simulink model "ctrl_student"  (R2014a)
settings: Solver=ode4  StartTime=0.0  StopTime=inf  FixedStep=0.01  RelTol=1e-3
undefined symbols (not defined in the file): M
libraries: marine_gnc x2
(part 2 of 2)

== system ctrl_student/Observer/nu_hat ==
  nu_hat : Inport
  Demux : Demux  Outputs=3
  r_hat : S-Function  Priority=3  FunctionName=NIVeriStandIO  Parameters=width dtype portnum stime stype btype  EnableBusSupport=off  mask(NI VeriStand Outport){portnum=3, width=-1, stime=-1, dtype=auto, stype=auto, btype=0}
      mask prompts: portnum "Port number:"; width "Port dimensions (-1 for dynamically sized):"; stime "Sample time (-1 for inherited):"; dtype "Data type:"; stype "Signal type:"; btype "Block type:"
      mask help: Use this outport on any level of nested subsystems to allow NI VeriStand software to map signals to it.
      mask init:
      | NIVeriStandIO_init;
      settings: CopyFcn=NIVeriStand_MDL_functions('', 'IO_copy');  DeleteFcn=NIVeriStand_MDL_functions('', 'IO_delete');  MoveFcn=set_param(gcb, 'Mask', 'on');
      mask Callback portnum: NIVeriStand_MDL_functions('', 'IO_setportnum');
      mask TypeOptions dtype: auto | double | single | int8 | uint8 | int16 | uint16 | int32 | uint32 | boolean
      mask Callback dtype: NIVeriStand_MDL_functions('', 'IO_booleansignal');
      mask TypeOptions stype: auto | real | complex
      mask Display:
      | patch([-x x], [-y y], [.90980 .81960 .32156]);
      | plot([xrad -x x xrad], [yrad -y y yrad]);
      | fprintf('NI Out%d', portnum);
  u_hat : S-Function  Priority=1  FunctionName=NIVeriStandIO  Parameters=width dtype portnum stime stype btype  EnableBusSupport=off  mask(NI VeriStand Outport){portnum=1, width=-1, stime=-1, dtype=auto, stype=auto, btype=0}
      mask prompts: portnum "Port number:"; width "Port dimensions (-1 for dynamically sized):"; stime "Sample time (-1 for inherited):"; dtype "Data type:"; stype "Signal type:"; btype "Block type:"
      mask help: Use this outport on any level of nested subsystems to allow NI VeriStand software to map signals to it.
      mask init:
      | NIVeriStandIO_init;
      settings: CopyFcn=NIVeriStand_MDL_functions('', 'IO_copy');  DeleteFcn=NIVeriStand_MDL_functions('', 'IO_delete');  MoveFcn=set_param(gcb, 'Mask', 'on');
      mask Callback portnum: NIVeriStand_MDL_functions('', 'IO_setportnum');
      mask TypeOptions dtype: auto | double | single | int8 | uint8 | int16 | uint16 | int32 | uint32 | boolean
      mask Callback dtype: NIVeriStand_MDL_functions('', 'IO_booleansignal');
      mask TypeOptions stype: auto | real | complex
      mask Display:
      | patch([-x x], [-y y], [.90980 .81960 .32156]);
      | plot([xrad -x x xrad], [yrad -y y yrad]);
      | fprintf('NI Out%d', portnum);
  v_hat : S-Function  Priority=2  FunctionName=NIVeriStandIO  Parameters=width dtype portnum stime stype btype  EnableBusSupport=off  mask(NI VeriStand Outport){portnum=2, width=-1, stime=-1, dtype=auto, stype=auto, btype=0}
      mask prompts: portnum "Port number:"; width "Port dimensions (-1 for dynamically sized):"; stime "Sample time (-1 for inherited):"; dtype "Data type:"; stype "Signal type:"; btype "Block type:"
      mask help: Use this outport on any level of nested subsystems to allow NI VeriStand software to map signals to it.
      mask init:
      | NIVeriStandIO_init;
      settings: CopyFcn=NIVeriStand_MDL_functions('', 'IO_copy');  DeleteFcn=NIVeriStand_MDL_functions('', 'IO_delete');  MoveFcn=set_param(gcb, 'Mask', 'on');
      mask Callback portnum: NIVeriStand_MDL_functions('', 'IO_setportnum');
      mask TypeOptions dtype: auto | double | single | int8 | uint8 | int16 | uint16 | int32 | uint32 | boolean
      mask Callback dtype: NIVeriStand_MDL_functions('', 'IO_booleansignal');
      mask TypeOptions stype: auto | real | complex
      mask Display:
      | patch([-x x], [-y y], [.90980 .81960 .32156]);
      | plot([xrad -x x xrad], [yrad -y y yrad]);
      | fprintf('NI Out%d', portnum);
  wires:
  Demux/1 -> u_hat/1
  Demux/2 -> v_hat/1
  Demux/3 -> r_hat/1
  nu_hat/1 -> Demux/1

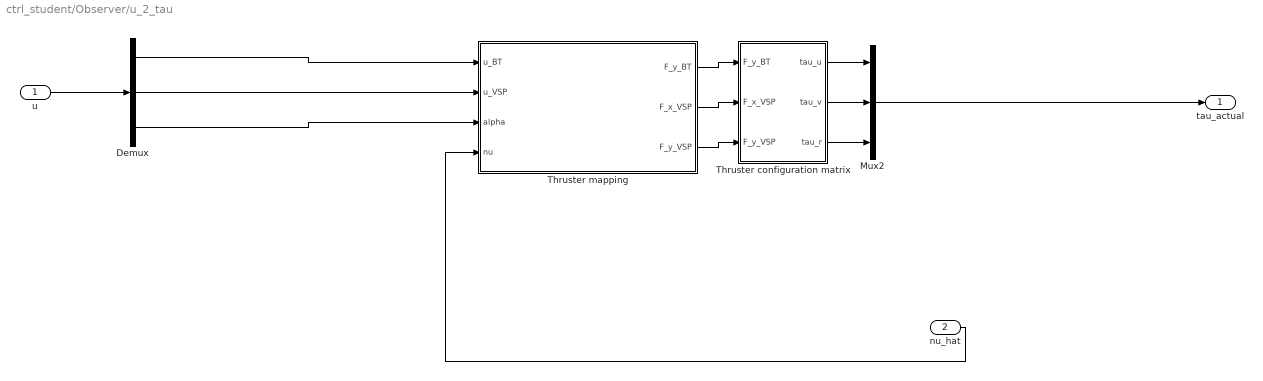
== system ctrl_student/Observer/u_2_tau ==
  u : Inport
  nu_hat : Inport  Port=2
  Demux : Demux  Outputs=3
  Mux2 : Mux  Inputs=3
  Thruster configuration matrix : MATLAB Function  TreatAsAtomicUnit=on
  Thruster mapping : Subsystem
  tau_actual : Outport
  wires:
  Thruster configuration matrix/1(tau_u) -> Mux2/1
  Thruster configuration matrix/2(tau_v) -> Mux2/2
  Thruster configuration matrix/3(tau_r) -> Mux2/3
  Thruster mapping/1(F_y_BT) -> Thruster configuration matrix/1(F_y_BT)
  Thruster mapping/2(F_x_VSP) -> Thruster configuration matrix/2(F_x_VSP)
  Thruster mapping/3(F_y_VSP) -> Thruster configuration matrix/3(F_y_VSP)
  nu_hat/1 -> Thruster mapping/4(nu)
  Mux2/1 -> tau_actual/1
  u/1 -> Demux/1
  Demux/1 -> Thruster mapping/1(u_BT)
  Demux/2 -> Thruster mapping/2(u_VSP)
  Demux/3 -> Thruster mapping/3(alpha)

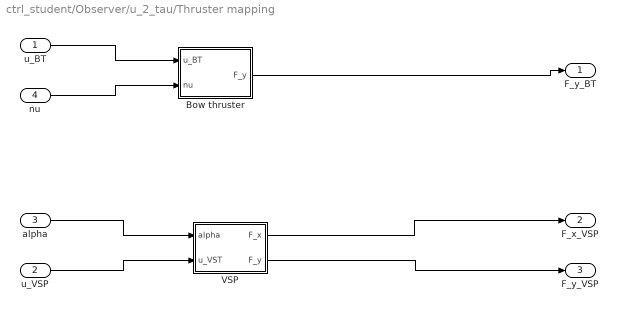
== system ctrl_student/Observer/u_2_tau/Thruster mapping ==
  u_BT : Inport
  u_VSP : Inport  Port=2
  alpha : Inport  Port=3
  nu : Inport  Port=4
  Bow thruster : MATLAB Function  TreatAsAtomicUnit=on
  VSP : MATLAB Function  TreatAsAtomicUnit=on
  F_y_BT : Outport
  F_x_VSP : Outport  Port=2
  F_y_VSP : Outport  Port=3
  wires:
  alpha/1 -> VSP/1(alpha)
  u_VSP/1 -> VSP/2(u_VST)
  nu/1 -> Bow thruster/2(nu)
  u_BT/1 -> Bow thruster/1(u_BT)
  Bow thruster/1(F_y) -> F_y_BT/1
  VSP/1(F_x) -> F_x_VSP/1
  VSP/2(F_y) -> F_y_VSP/1

== matlab function ctrl_student/Thrust allocation ==
  data: X_d input; Y_d input; u_BT output; N_d input; u_VSP output; alpha_VSP output; VSP_on input; omega_VSP output
function [u_BT,u_VSP,alpha_VSP,omega_VSP]= fcn(X_d,Y_d,N_d, VSP_on)

% Forces and moments vector
tau = [X_d
       Y_d
       N_d];

% Extended thrust configuration matrix
l_VSP = -0.4575;
l_BT  = 0.3875;
T = [1 0     0
     0 1     1
     0 l_VSP l_BT];

% Extended thrust coefficient matrix
F_max_VSP = 1.165;
F_max_BT  = 2.629;
K = [F_max_VSP 0         0
     0         F_max_VSP 0
     0         0         F_max_BT];

% tau = T*K*u inverse
u = K\(T\tau);

u_BT      = u(3);

u_VSP_x   = u(1);
u_VSP_y   = u(2);
u_VSP     = sqrt(u_VSP_x^2 + u_VSP_y^2);
alpha_VSP = atan2(u_VSP_y,u_VSP_x);

if VSP_on
    omega_VSP = 0.3;
else
    omega_VSP = 0;
end

== matlab function ctrl_student/control limit checking ==
  data: u input; fault output
function fault= fcn(u)
u_BT       = u(1);
u_VSP1     = u(2);
u_VSP2     = u(3);
alpha_VSP1 = u(4);
alpha_VSP2 = u(5);
omega_VSP1 = u(6);
omega_VSP2 = u(7);

OK = -1  <= u_BT       & u_BT       <= 1  & ...
     0   <= u_VSP1     & u_VSP1     <= 1  & ...
     0   <= u_VSP1     & u_VSP1     <= 2  & ...
     -pi <= alpha_VSP1 & alpha_VSP1 <= pi & ...
     -pi <= alpha_VSP2 & alpha_VSP2 <= pi & ...
     -1  <= omega_VSP1 & omega_VSP1 <= 1  & ...
     -1  <= omega_VSP2 & omega_VSP2 <= 1  ;
 
fault = ~OK;

== matlab function ctrl_student/Derivative filter/Differentiate and filter1 ==
  data: nu input; nu_dot output; nu_prev input; nu_dot_prev input
function nu_dot = fcn(nu,nu_prev,nu_dot_prev)

% derivative
h = 0.01;
nu_dot = (nu-nu_prev)./h;

% filter
a = 0.01;
nu_dot = a*nu_dot + (1-a)*nu_dot_prev;

== matlab function ctrl_student/Observer/u_2_tau/Thruster configuration matrix ==
  data: F_y_BT input; tau_u output; F_x_VSP input; F_y_VSP input; tau_v output; tau_r output
function [tau_u, tau_v, tau_r] = fcn(F_y_BT, F_x_VSP, F_y_VSP)
%#codegen

L_VSP = -0.4575;
L_BT = 0.3875;

u = [F_x_VSP;F_y_VSP;F_y_BT];

T = [1 0 0;
     0 1 1;
     0 L_VSP L_BT];

tau = T*u; 

tau_u = tau(1);
tau_v = tau(2);
tau_r = tau(3);

== matlab function ctrl_student/Observer/u_2_tau/Thruster mapping/Bow thruster ==
  data: u_BT input; F_y output; nu input
function F_y = fcn(u_BT,nu)
%#codegen
u = nu(1);
% Thruster characteristics
if u_BT > 0.0879
    a =       2.515;
    b =      0.1174;
    c =      -2.807;
    d =      -1.131;
    y0 = a*exp(b*u_BT) + c*exp(d*u_BT);
elseif u_BT < -0.059
    a =        -548;
    b =       0.193;
    c =       548.2;
    d =      0.1992;
    y0 = a*exp(b*u_BT) + c*exp(d*u_BT);
else
    y0 = 0;
end
% Thruster losses due to forward speed
a0 =      0.7561;
a1 =      0.3075;
b1 =      -10.22;
c1 =       2.947;
F_y = y0*(a0 + a1*atan(b1*u +c1))/1.1385;

== matlab function ctrl_student/Observer/D(nu)*nu ==
  data: nu_hat input; D_nl output
function D_nl = fcn(nu_hat)
%#codegen
u = nu_hat(1);
v = nu_hat(2);
r = nu_hat(3);

D_NL = ctrl_student_observer_D(u,v,r);

D_nl =D_NL*nu_hat;

== matlab function ctrl_student/Observer/C(nu)*nu ==
  data: nu_hat input; C_nl output
function C_nl = fcn(nu_hat)
%#codegen
u = nu_hat(1);
v = nu_hat(2);
r = nu_hat(3);

C_NL = ctrl_student_observer_C(u,v,r);

C_nl =C_NL*nu_hat;

== matlab function ctrl_student/Observer/u_2_tau/Thruster mapping/VSP ==
  data: alpha input; F_x output; u_VST input; F_y output
function [ F_x , F_y ] = fcn(alpha,u_VST)
%#codegen
% Calculating the force in x-direction
a1 =       1.107  ;
b1 =       1.001  ;
c1 =       1.564  ;
a2 =      0.3471 ;
b2 =      0.1397 ;
c2 =      -1.599  ;
a3 =      0.1558 ;
b3 =       1.993  ;
c3 =       1.886  ;
a4 =      0.1599 ;
b4 =       0.218  ;
c4 =       1.513  ;
a5 =     0.08237 ;
b5 =       2.986  ;
c5 =      -1.601  ;
a6 =     0.04641 ;
b6 =       3.964  ;
c6 =       1.738  ;
F_x =   u_VST*( a1*sin(b1*alpha+c1) + ...
                a2*sin(b2*alpha+c2) + ...
                a3*sin(b3*alpha+c3) + ...
                a4*sin(b4*alpha+c4) + ...
                a5*sin(b5*alpha+c5) + ...
                a6*sin(b6*alpha+c6) );
% Calculating the force in y-direction
a1 =      0.7936 ;
b1 =       1.001  ;
c1 =     0.01605;
a2 =      0.2112 ;
b2 =       1.997  ;
c2 =     0.03229;
a3 =     0.07608;
b3 =       2.991  ;
c3 =       2.986  ;
a4 =     0.04817;
b4 =       3.999  ;
c4 =     -0.8668 ;
a5 =     0.01757;
b5 =       4.904  ;
c5 =      -2.622 ;
a6 =    -0.02089;
b6 =       5.068  ;
c6 =      0.2548 ;
F_y =   u_VST*( a1*sin(b1*alpha+c1) + ...
                a2*sin(b2*alpha+c2) + ...
                a3*sin(b3*alpha+c3) + ...
                a4*sin(b4*alpha+c4) + ...
                a5*sin(b5*alpha+c5) + ...
                a6*sin(b6*alpha+c6));

== matlab function ctrl_student/Observer/MATLAB Function ==
  data: K_p output; K_p1 input
function K_p = fcn(K_p1)
%#codegen

K_p = diag(K_p1);

== matlab function ctrl_student/Observer/MATLAB Function1 ==
  data: K_i output; K_i1 input
function K_i = fcn(K_i1)
%#codegen

K_i = diag(K_i1);

== matlab function ctrl_student/Observer/MATLAB Function2 ==
  data: K_d output; K_d1 input
function K_d = fcn(K_d1)
%#codegen

K_d = diag(K_d1);

== matlab function ctrl_student/Derivative filter/Low pass filter ==
  data: a input; eta_filtered output; eta input; eta_filtered_prev input
function eta_filtered = fcn(a,eta,eta_filtered_prev)

eta_filtered = a*eta + (1-a)*eta_filtered_prev;

== matlab function ctrl_student/Derivative filter/Discrete derivative ==
  data: h input; eta_dot output; eta input; eta_prev input
function eta_dot = fcn(h,eta,eta_prev)

eta_dot = (eta-eta_prev)./h;

== matlab function ctrl_student/Derivative filter/Low pass filter 2 ==
  data: a input; eta_dot_filtered output; eta_dot input; eta_dot_filtered_prev input
function eta_dot_filtered = fcn(a,eta_dot,eta_dot_filtered_prev)

eta_dot_filtered = a*eta_dot + (1-a)*eta_dot_filtered_prev;

== matlab function ctrl_student/Derivative filter/Rotation matrix ==
  data: eta_dot input; nu output; psi input
function nu = fcn(eta_dot,psi)

R_inv = [cos(psi)  sin(psi) 0
         -sin(psi) cos(psi) 0
         0         0        1];
nu = R_inv*eta_dot;
